simulink model "Program_1_SIR_Italy 2"  (R2020a)
settings: Solver=FixedStepAuto  StartTime=0.0  StopTime=180  FixedStep=0.001  RelTol=1e-9  AbsTol=1e-9
undefined symbols (not defined in the file): a, beta, gamma1, gamma2, gamma3, I0, P, R0, st3, zeta1, zeta2, zeta3
libraries: fuzblock x3
settings Model: OrderedModelArguments=off  Creator=ismae  LastModifiedBy=ismae
settings SolverCC: SolverResetMethod=Robust

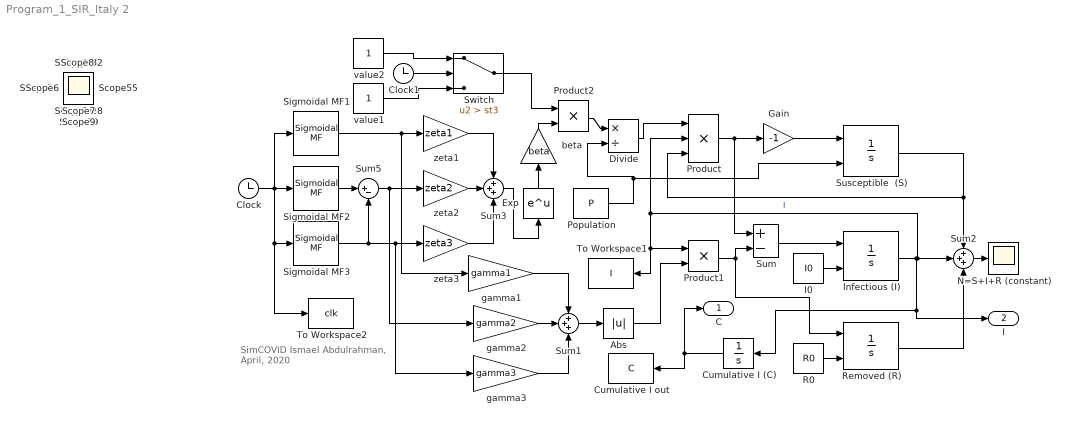
== system Program_1_SIR_Italy 2 ==
  note: SimCOVID
      | Ismael Abdulrahman, April, 2020
  Abs : Abs
  Clock : Clock
  Clock1 : Clock
  Cumulative I (C) : Integrator
  Cumulative I out : ToWorkspace  VariableName=C  SampleTime=-1
      settings: Save2DSignal=2-D array (concatenate along first dimension)
  Divide : Product  Inputs=*/
  Exp : Math  SaturateOnIntegerOverflow=on
  Gain : Gain  Gain=-1
  I0 : Constant  Value=I0
  Infectious (I) : Integrator  InitialConditionSource=external
  N=S+I+R (constant) : Scope
  Population : Constant  Value=P
  Product : Product  Inputs=3
  Product1 : Product
  Product2 : Product
  R0 : Constant  Value=R0
  Removed (R) : Integrator  InitialConditionSource=external
  Sigmoidal MF1 : fuzblock/Membership  Functions/Sigmoidal MF  a=-a  c=st1
      settings: SourceProductBaseCode=FL
  Sigmoidal MF2 : fuzblock/Membership  Functions/Sigmoidal MF  a=a  c=st1
      settings: SourceProductBaseCode=FL
  Sigmoidal MF3 : fuzblock/Membership  Functions/Sigmoidal MF  a=a  c=st2
      settings: SourceProductBaseCode=FL
  Sum : Sum  Inputs=+-
  Sum1 : Sum  Inputs=+++
  Sum2 : Sum  Inputs=+++
  Sum3 : Sum  Inputs=+++
  Sum5 : Sum  Inputs=|+-
  Susceptible  (S) : Integrator  InitialConditionSource=external  InitialCondition=10000
  Switch : Switch  Criteria=u2 > Threshold  Threshold=st3
  To Workspace1 : ToWorkspace  VariableName=I  SampleTime=-1
      settings: Save2DSignal=2-D array (concatenate along first dimension)
  To Workspace2 : ToWorkspace  VariableName=clk  SampleTime=-1
      settings: Save2DSignal=2-D array (concatenate along first dimension)
  beta : Gain  Gain=beta
  gamma1 : Gain  Gain=gamma1
  gamma2 : Gain  Gain=gamma2
  gamma3 : Gain  Gain=gamma3
  value1 : Constant
  value2 : Constant
  zeta1 : Gain  Gain=zeta1
  zeta2 : Gain  Gain=zeta2
  zeta3 : Gain  Gain=zeta3
  C : Outport
  I : Outport  Port=2
  Scope{,1..32} (33 alike) : Scope
  wires:
  Product/1 -> Gain/1, Sum/1
  Divide/1 -> Product/1
  Sum/1 -> Infectious (I)/1
  I0/1 -> Infectious (I)/2
  Population/1 -> Susceptible  (S)/2, Divide/2
  Sum2/1 -> N=S+I+R (constant)/1
  R0/1 -> Removed (R)/2
  Product1/1 -> Removed (R)/1, Sum/2
  zeta3/1 -> Sum3/3
  zeta2/1 -> Sum3/2
  zeta1/1 -> Sum3/1
  Susceptible  (S)/1 -> Product/3, Sum2/1
  Gain/1 -> Susceptible  (S)/1
  Removed (R)/1 -> Sum2/3
  Cumulative I (C)/1 -> Cumulative I out/1, C/1
  Sum3/1 -> Exp/1
  Exp/1 -> beta/1
  Sum1/1 -> Abs/1
  Sigmoidal MF1/1 -> gamma1/1, zeta1/1
  Sigmoidal MF2/1 -> Sum5/1
  gamma1/1 -> Sum1/1
  Sigmoidal MF3/1 -> gamma3/1, zeta3/1, Sum5/2
  Sum5/1 -> gamma2/1, zeta2/1
  gamma3/1 -> Sum1/3
  gamma2/1 -> Sum1/2
  Clock/1 -> Sigmoidal MF1/1, Sigmoidal MF2/1, Sigmoidal MF3/1, To Workspace2/1
  beta/1 -> Product2/2
  Product2/1 -> Divide/1
  Clock1/1 -> Switch/2
  Switch/1 -> Product2/1
  value2/1 -> Switch/1
  value1/1 -> Switch/3
  Infectious (I)/1 -> Product1/1, To Workspace1/1, Product/2, Sum2/2, I/1, Cumulative I (C)/1  "I"
  Abs/1 -> Product1/2
